simulink model "test_sdr_mimo"  (R2020a)
settings: Solver=FixedStepAuto  StartTime=0.0  StopTime=inf  FixedStep=system.step  RelTol=1e-3
undefined symbols (not defined in the file): SDR
libraries: dspsrcs4 x2, dspmathops x1, commanabbnd3 x1
settings Model: Creator=jose_  LastModifiedBy=jose_

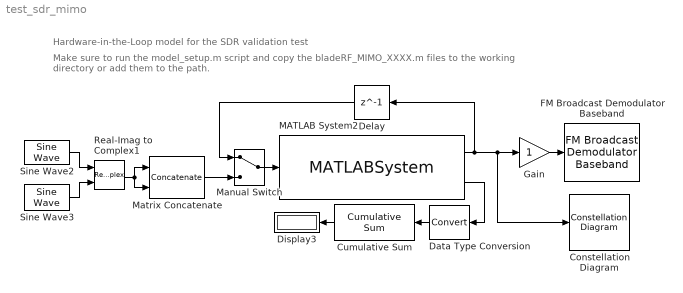
== system test_sdr_mimo ==
  note: Make sure to run the model_setup.m script and copy the bladeRF_MIMO_XXXX.m files to the working directory or add them to the path.
  note: Hardware-in-the-Loop model for the SDR validation test
  Constellation Diagram : ConstellationDiagram
  Cumulative Sum : dspmathops/Cumulative Sum  dim=Channels (running sum)  reset_popup=None  roundingMode=Floor  overflowMode=off  outputDataTypeStr=Inherit: Same as accumulator  outputMin=[]  outputMax=[]  outputLastDataTypeStr=Inherit: Same as accumulator
  Data Type Conversion : DataTypeConversion
  Delay : Delay  DelayLength=1
  Display3 : Display
  FM Broadcast Demodulator Baseband : commanabbnd3/FM Broadcast Demodulator Baseband  SampleRate=SDR.samplerate  FrequencyDeviation=75e3  FilterTimeConstant=75e-6  AudioSampleRate=48000  PlaySound=on  BufferSize=SDR.samples_per_step  Stereo=off  RBDS=off  RBDSSamplesPerSymbol=10  RBDSCostasLoop=off  SimulateUsing=Code generation
      settings: SourceProductBaseCode=CM
  Gain : Gain
  MATLAB System2 : MATLABSystem  System=bladeRF_MIMO_Simulink  loopback_mode=None  xb200=off  SimulateUsing=Interpreted execution  enable_rx=on  enable_overrun=on  rx_frequency=system.freq  rx_samplerate=SDR.samplerate  rx_bandwidth=1.5  rx_gain=SDR.rx_gain  enable_rx_biastee=off  rx_agc=SLOW  rx_num_buffers=SDR.stream.n_buffers  rx_num_transfers=SDR.stream.n_transfers  rx_buf_size=SDR.stream.buffer_size  rx_timeout_ms=SDR.stream.timeout  rx_step_size=SDR.samples_per_step  enable_tx=on  enable_underrun=off  tx_frequency=system.freq  tx_samplerate=SDR.samplerate  tx_bandwidth=1.5  tx_gain=SDR.tx_gain  enable_tx_biastee=off  tx_num_buffers=SDR.stream.n_buffers  tx_num_transfers=SDR.stream.n_transfers  tx_buf_size=SDR.stream.buffer_size  tx_timeout_ms=SDR.stream.timeout  tx_step_size=SDR.samples_per_step  verbosity=Verbose
      mask Type: bladeRF_MIMO_Simulink
      mask Display:
      | disp(['Nuand' char(10) 'bladeRF 2.0' char(10) 'MIMO']);
      | port_label('input',1,'TX Samples');
      | port_label('output',1,'RX Samples');
      | port_label('output',2,'RX Overrun');
  Manual Switch : ManualSwitch
  Matrix Concatenate : Concatenate  Mode=Multidimensional array  ConcatenateDimension=2
  Real-Imag to Complex1 : RealImagToComplex
  Sine Wave2 : dspsrcs4/Sine Wave  Amplitude=1  Frequency=100  Phase=0  SampleMode=Discrete  OutComplex=Real  CompMethod=Table lookup  TableSize=Speed  SampleTime=1/SDR.samplerate  SamplesPerFrame=SDR.samples_per_step  ResetState=Restart at time zero  OutputFrames=off  dataType=double  wordLen=16  udDataType=sfix(16)  fracBitsMode=Best precision  numFracBits=15  OutDataTypeStr=double  LastOutDataTypeStr=double
  Sine Wave3 : dspsrcs4/Sine Wave  Amplitude=0.6  Frequency=100  Phase=pi/2  SampleMode=Discrete  OutComplex=Real  CompMethod=Table lookup  TableSize=Speed  SampleTime=1/SDR.samplerate  SamplesPerFrame=SDR.samples_per_step  ResetState=Restart at time zero  OutputFrames=off  dataType=double  wordLen=16  udDataType=sfix(16)  fracBitsMode=Best precision  numFracBits=15  OutDataTypeStr=double  LastOutDataTypeStr=double
  wires:
  Data Type Conversion/1 -> Cumulative Sum/1
  Cumulative Sum/1 -> Display3/1
  MATLAB System2/2 -> Data Type Conversion/1
  MATLAB System2/1 -> Constellation Diagram/1, Gain/1, Delay/1
  Gain/1 -> FM Broadcast Demodulator Baseband/1
  Sine Wave3/1 -> Real-Imag to Complex1/2
  Sine Wave2/1 -> Real-Imag to Complex1/1
  Real-Imag to Complex1/1 -> Matrix Concatenate/2, Matrix Concatenate/1
  Manual Switch/1 -> MATLAB System2/1
  Matrix Concatenate/1 -> Manual Switch/2
  Delay/1 -> Manual Switch/1
